simulink model "SIMULINKLINEARNI"  (R2020b)
settings: Solver=VariableStepAuto  StartTime=0.0  StopTime=10.0  RelTol=1e-3
values from neighbouring files (symbols this model uses):
  b1 = 0.0050134512    [I_PD.m]    (also in LQR.m = 0.05; PODACI.m = 0.05; Untitled2.m)
  b2 = 45    [LQR.m]    (also in PODACI.m)
  c = 0.03    [LQR.m]    (also in PODACI.m)
  d = 0.062    [LQR.m]    (also in PODACI.m)
  g = 9.81    [LQR.m]    (also in PODACI.m)
  M = 1.2    [LQR.m]    (also in PODACI.m)
  m = 0.3    [LQR.m]    (also in PODACI.m)
settings Model: Creator=Toni  LastModifiedBy=Toni

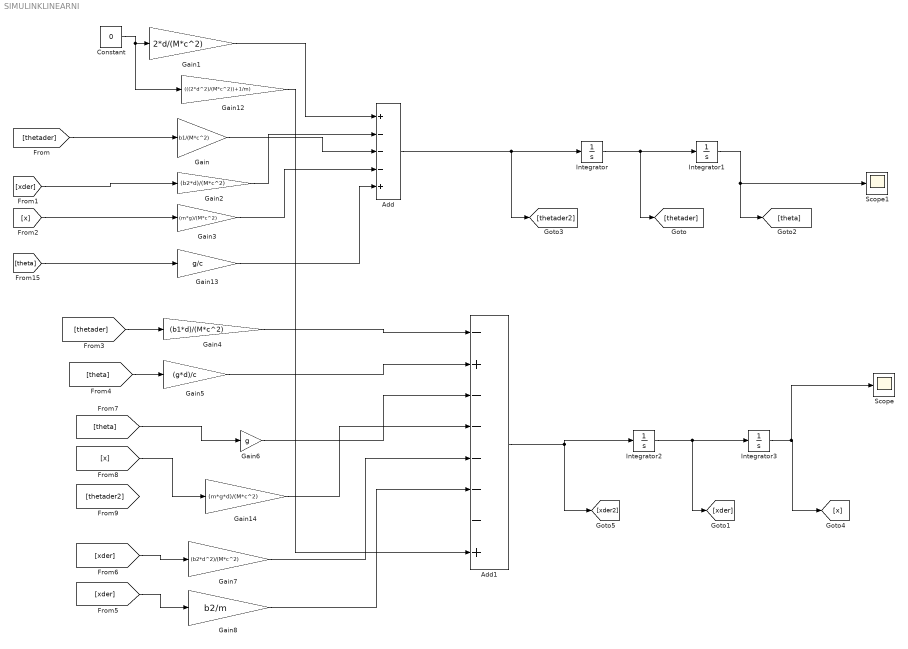
== system SIMULINKLINEARNI ==
  Add : Sum  Inputs=+---+
  Add1 : Sum  Inputs=-+-----+
  Constant : Constant  Value=0
  Gain : Gain  Gain=b1/(M*c^2)
  Gain1 : Gain  Gain=2*d/(M*c^2)
  Gain12 : Gain  Gain=(((2*d^2)/(M*c^2))+1/m)
  Gain13 : Gain  Gain=g/c
  Gain14 : Gain  Gain=(m*g*d)/(M*c^2)
  Gain2 : Gain  Gain=(b2*d)/(M*c^2)
  Gain3 : Gain  Gain=(m*g)/(M*c^2)
  Gain4 : Gain  Gain=(b1*d)/(M*c^2)
  Gain5 : Gain  Gain=(g*d)/c
  Gain6 : Gain  Gain=g
  Gain7 : Gain  Gain=(b2*d^2)/(M*c^2)
  Gain8 : Gain  Gain=b2/m
  Integrator{,1..3} (4 alike) : Integrator
  Scope : Scope
  Scope1 : Scope
  wires:
  Gain5/1 -> Add1/2
  [x] -> Gain14/1
  Integrator3/1 -> Scope/1, [x]
  Gain6/1 -> Add1/3
  Integrator2/1 -> [xder], Integrator3/1
  Integrator/1 -> [thetader], Integrator1/1
  Gain4/1 -> Add1/1
  Add1/1 -> Integrator2/1, [xder2]
  [xder] -> Gain7/1
  [x] -> Gain3/1
  Integrator1/1 -> Scope1/1, [theta]
  [thetader] -> Gain4/1
  Gain12/1 -> Add1/8
  [theta] -> Gain5/1
  [xder] -> Gain2/1
  [thetader] -> Gain/1
  Add/1 -> [thetader2], Integrator/1
  [theta] -> Gain6/1
  Constant/1 -> Gain12/1, Gain1/1
  Gain1/1 -> Add/1
  Gain2/1 -> Add/2
  Gain/1 -> Add/3
  Gain3/1 -> Add/4
  [theta] -> Gain13/1
  Gain13/1 -> Add/5
  Gain14/1 -> Add1/4
  [xder] -> Gain8/1
  Gain7/1 -> Add1/5
  Gain8/1 -> Add1/6
